simulink model "model"  (R2016a)
settings: Solver=VariableStepAuto  StartTime=0.0  StopTime=10  RelTol=1e-3
values from neighbouring files (symbols this model uses):
  delta_a = U_trim(2)    [test_model.m]
  delta_e = U_trim(1)    [test_model.m]
  delta_r = U_trim(3)    [test_model.m]
  delta_t = U_trim(4)    [test_model.m]
undefined symbols (not defined in the file or in its folder): X_trim
settings Model: Creator=andreanv  LastModifiedBy=andreanv

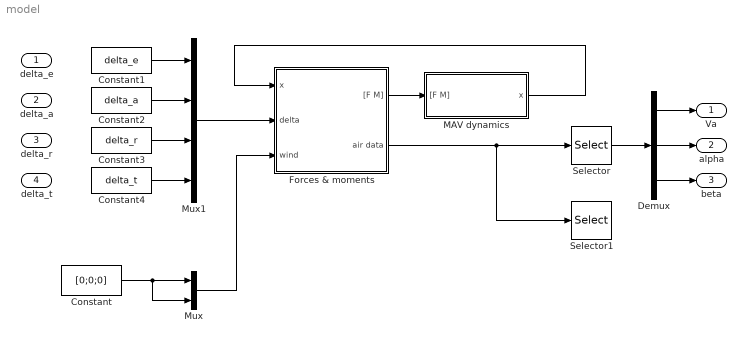
== system model ==
  delta_e : Inport
  delta_a : Inport  Port=2
  delta_r : Inport  Port=3
  delta_t : Inport  Port=4
  Constant : Constant  Value=[0;0;0]
  Constant1 : Constant  Value=delta_e
  Constant2 : Constant  Value=delta_a
  Constant3 : Constant  Value=delta_r
  Constant4 : Constant  Value=delta_t
  Demux : Demux  Outputs=3
  Forces & moments : Subsystem
  MAV dynamics : Subsystem
  Mux : Mux  Inputs=2
  Mux1 : Mux
  Selector : Selector  InputPortWidth=6  IndexOptions=Index vector (dialog)  Indices=[1 2 3]  OutputSizes=1
  Selector1 : Selector  InputPortWidth=6  IndexOptions=Index vector (dialog)  Indices=[4 5 6]  OutputSizes=1
  Va : Outport
  alpha : Outport  Port=2
  beta : Outport  Port=3
  wires:
  Forces & moments/2(air data) -> Selector1/1, Selector/1
  Demux/3 -> beta/1
  Demux/2 -> alpha/1
  Demux/1 -> Va/1
  Mux/1 -> Forces & moments/3(wind)
  Constant/1 -> Mux/2, Mux/1
  MAV dynamics/1(x) -> Forces & moments/1(x)
  Mux1/1 -> Forces & moments/2(delta)
  Forces & moments/1("[F M]") -> MAV dynamics/1("[F M]")
  Selector/1 -> Demux/1
  Constant1/1 -> Mux1/1
  Constant2/1 -> Mux1/2
  Constant3/1 -> Mux1/3
  Constant4/1 -> Mux1/4

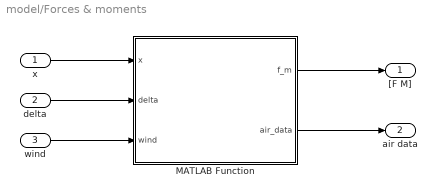
== system model/Forces & moments ==
  x : Inport
  delta : Inport  Port=2
  wind : Inport  Port=3
  MATLAB Function : MATLAB Function  TreatAsAtomicUnit=on
  "[F M]" : Outport
  air data : Outport  Port=2
  wires:
  x/1 -> MATLAB Function/1(x)
  delta/1 -> MATLAB Function/2(delta)
  wind/1 -> MATLAB Function/3(wind)
  MATLAB Function/1(f_m) -> "[F M]"/1
  MATLAB Function/2(air_data) -> air data/1

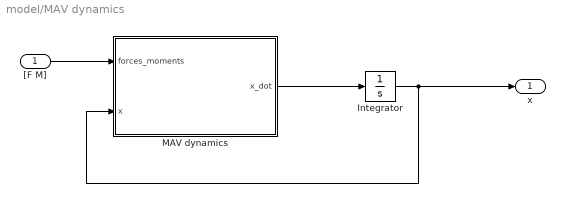
== system model/MAV dynamics ==
  "[F M]" : Inport  OutMin=[6]  OutMax=[6]
  Integrator : Integrator  InitialCondition=X_trim
  MAV dynamics : MATLAB Function  TreatAsAtomicUnit=on
  x : Outport
  wires:
  Integrator/1 -> x/1, MAV dynamics/2(x)
  "[F M]"/1 -> MAV dynamics/1(forces_moments)
  MAV dynamics/1(x_dot) -> Integrator/1

== matlab function model/MAV dynamics/MAV dynamics ==
  data: forces_moments input; x_dot output; x input; P parameter
function x_dot = fcn(forces_moments, x, P)

    x_dot = mav_dynamics(forces_moments, x, P);
    
end

== matlab function model/Forces & moments/MATLAB Function ==
  data: x input; f_m output; delta input; wind input; air_data output; P parameter
function [f_m, air_data] = fcn(x, delta, wind, P)

    output = forces_moments(x, delta, wind, P);
    
    f_m = output(1:6);
    air_data = output(7:12);

end
